simulink subsystem "filtro_LP_temperatura"  (R2023b)
settings: Solver=VariableStepAuto  StartTime=0.0  StopTime=10.0  RelTol=1e-3
undefined symbols (not defined in the file or in its folder): tau
settings Model: Creator=nicol  LastModifiedBy=nicol

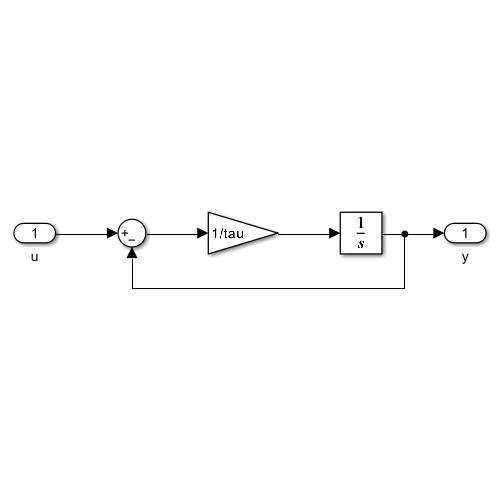
[thumbnail: Simulink's stored preview of the top-level diagram]
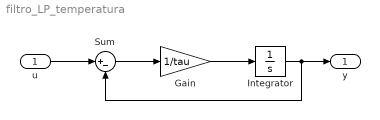
== system filtro_LP_temperatura ==
  u : Inport
  Gain : Gain  Gain=1/tau
  Integrator : Integrator
  Sum : Sum  Inputs=|+-
  y : Outport
  wires:
  Integrator/1 -> Sum/2, y/1
  Gain/1 -> Integrator/1
  Sum/1 -> Gain/1
  u/1 -> Sum/1
